simulink model "nsdynamic"  (R2021b)
settings: Solver=ode4  StartTime=0.0  StopTime=10.0  RelTol=1e-3
InitFcn:
  | initialization
undefined symbols (not defined in the file or in its folder): dynNS, trajectory
settings Model: Creator=AzamaoZ  LastModifiedBy=AzamaoZ

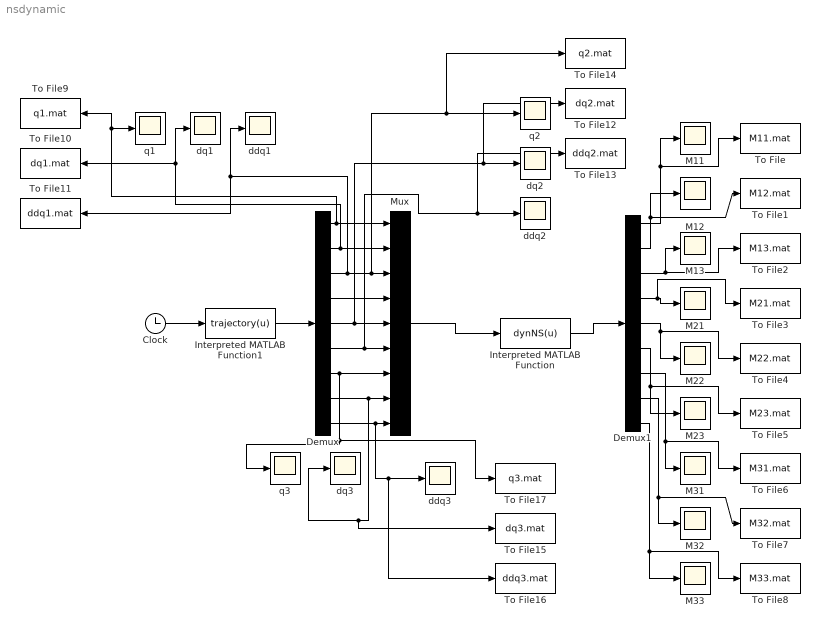
== system nsdynamic ==
  Clock : Clock
  Demux : Demux  Outputs=9
  Demux1 : Demux  Outputs=9
  Interpreted MATLAB Function : MATLABFcn  MATLABFcn=dynNS(u)  OutputDimensions=9
  Interpreted MATLAB Function1 : MATLABFcn  MATLABFcn=trajectory(u)
  M{11..13,21..23,31..33} (9 alike) : Scope
  Mux : Mux  Inputs=9
  To File : ToFile  Filename=M11.mat  MatrixName=M11  SaveFormat=Timeseries
  To File1 : ToFile  Filename=M12.mat  MatrixName=M12  SaveFormat=Timeseries
  To File10 : ToFile  Filename=dq1.mat  MatrixName=dq1  SaveFormat=Timeseries
  To File11 : ToFile  Filename=ddq1.mat  MatrixName=ddq1  SaveFormat=Timeseries
  To File12 : ToFile  Filename=dq2.mat  MatrixName=dq2  SaveFormat=Timeseries
  To File13 : ToFile  Filename=ddq2.mat  MatrixName=ddq2  SaveFormat=Timeseries
  To File14 : ToFile  Filename=q2.mat  MatrixName=q2  SaveFormat=Timeseries
  To File15 : ToFile  Filename=dq3.mat  MatrixName=dq3  SaveFormat=Timeseries
  To File16 : ToFile  Filename=ddq3.mat  MatrixName=ddq3  SaveFormat=Timeseries
  To File17 : ToFile  Filename=q3.mat  MatrixName=q3  SaveFormat=Timeseries
  To File2 : ToFile  Filename=M13.mat  MatrixName=M13  SaveFormat=Timeseries
  To File3 : ToFile  Filename=M21.mat  MatrixName=M21  SaveFormat=Timeseries
  To File4 : ToFile  Filename=M22.mat  MatrixName=M22  SaveFormat=Timeseries
  To File5 : ToFile  Filename=M23.mat  MatrixName=M23  SaveFormat=Timeseries
  To File6 : ToFile  Filename=M31.mat  MatrixName=M31  SaveFormat=Timeseries
  To File7 : ToFile  Filename=M32.mat  MatrixName=M32  SaveFormat=Timeseries
  To File8 : ToFile  Filename=M33.mat  MatrixName=M33  SaveFormat=Timeseries
  To File9 : ToFile  Filename=q1.mat  MatrixName=q1  SaveFormat=Timeseries
  ddq1 : Scope
  ddq2 : Scope
  ddq3 : Scope
  dq1 : Scope
  dq2 : Scope
  dq3 : Scope
  q1 : Scope
  q2 : Scope
  q3 : Scope
  wires:
  Interpreted MATLAB Function/1 -> Demux1/1
  Clock/1 -> Interpreted MATLAB Function1/1
  Demux1/1 -> M11/1, To File/1
  Demux1/8 -> To File7/1, M32/1
  Demux1/2 -> M12/1, To File1/1
  Mux/1 -> Interpreted MATLAB Function/1
  Interpreted MATLAB Function1/1 -> Demux/1
  Demux/7 -> To File17/1, q3/1, Mux/7
  Demux1/7 -> To File6/1, M31/1
  Demux/6 -> To File13/1, ddq2/1, Mux/6
  Demux1/9 -> To File8/1, M33/1
  Demux/1 -> To File9/1, q1/1, Mux/1
  Demux/9 -> To File16/1, ddq3/1, Mux/9
  Demux/4 -> Mux/4
  Demux/5 -> To File12/1, dq2/1, Mux/5
  Demux/3 -> ddq1/1, To File11/1, To File14/1, q2/1, Mux/3
  Demux1/4 -> To File3/1, M21/1
  Demux/2 -> To File10/1, dq1/1, Mux/2
  Demux1/6 -> M23/1, To File5/1
  Demux/8 -> To File15/1, dq3/1, Mux/8
  Demux1/5 -> M22/1, To File4/1
  Demux1/3 -> M13/1, To File2/1
